simulink library "ddm"  (R2021b)
settings: Solver=VariableStepAuto  StartTime=0.0  StopTime=10.0  RelTol=1e-3
undefined symbols (not defined in the file or in its folder): ADDM_FrTMTqDev_X_Nm, ADDM_RrTMTqDev_X_Nm, ENUM_ADASACCSTA_ERROR, ENUM_ADASACCSTA_OFF, ENUM_ADASACCSTA_STANDBY, ENUM_ALLOWMOV_ALLOWREADY, ENUM_APS, ENUM_BRKSTA_ERROR, ENUM_BRKSTA_OFF, ENUM_BRKSTA_ON, ENUM_BRKSW_INVALID, ENUM_BRKSW_OFF, ENUM_BRKSW_ON, ENUM_CHGPREACTERRSTA_OBCPRE, ENUM_DCDCFAULTSTA_ANYFAULTLV1, ENUM_DCDCFAULTSTA_ANYFAULTLV2, ENUM_DRIVETRAIN_AWD, ENUM_DRIVETRAIN_FWD, ENUM_DRIVETRAIN_RWD, ENUM_EDUDRTSTA_NORMAL, ENUM_EPBSTA_APPLIED, ENUM_EPBSTA_RELEASED, ENUM_GEARACTUALPOSN_INVALID, ENUM_GEARACTUALPOSN_P, ENUM_HVBATTREADYPRE_READY, ENUM_MCUWARN_LV0, ENUM_MCUWARN_LV1, ENUM_MCUWARN_LV2, ENUM_MCUWARN_LV3, ENUM_MCUWARN_NOERROR, ENUM_OBCFAULTSTA_ANYFAULT, ENUM_PAS_R2F2, ENUM_PDFAULT_BATTPDFAIL, ENUM_PDFAULT_DCDCDISABLE, ENUM_PDFAULT_MCUDISABLE, ENUM_PDFAULT_MCUDISCHRG, ENUM_POWERSTA_OFF, ENUM_POWERSTA_ON, ENUM_POWERSTA_READY, ENUM_POWERSTA_STANDBY, ENUM_PRESSINDI_LOW, ENUM_PUFAULT_BATTUPFAIL, ENUM_PUFAULT_DCDCENABLEFAIL, ENUM_PUFAULT_PRECHRGCHKFAIL, ENUM_PUFAULT_SAFETYCHKFAIL, ENUM_PUSTATE_COMPLETED, ENUM_PWRSTASW_OFF, ENUM_PWRSTASW_OFFA, ENUM_PWRSTASW_OFFCHVCHRG, ENUM_PWRSTASW_OFFCLVCHRG, ENUM_PWRSTASW_ON, ENUM_PWRSTASW_ONHVCHRG, ENUM_PWRSTASW_READY, ENUM_PWRSTASW_STANDBY, ENUM_SHIFTCOMMAND_P, ENUM_SHIFTERERRSTA_PBUTTONFAILURE, ENUM_VEHMALFUNLV_2ND, ENUM_VEHMALFUNLV_3RD, ENUM_VEHMALFUNLV_4TH, ENUM_VEHMALFUNLV_NORMAL ... (+459)
libraries: hcu_lib x521, $bdroot x5, simulink x3
(part 8 of 25)

== system ddm/DDM/DDM/APM/Subsystem9 ==
  USSSta_flg : Inport
  VPMM_SysPwrSta_enum : Inport  Port=2
  VAPM_SNSRLayout_enum : Inport  Port=3
  Constant1 : Constant  Value=ENUM_PWRSTASW_READY
  Constant17 : Constant  Value=ENUM_PWRSTASW_READY
  Constant2 : Constant  Value=ENUM_PWRSTASW_ON
  Constant25 : Constant  Value=FALSE
  Constant3 : Constant  Value=ENUM_PWRSTASW_ON
  Constant5 : Constant  Value=ENUM_APS
  Equal{1..3,5..6} (5 alike) : RelationalOperator  Operator===  OutDataTypeStr=boolean  RndMeth=Simplest
  Logical Operator1 : Logic  Operator=NOT  AllPortsSameDT=off  OutDataTypeStr=boolean
  Logical Operator13 : Logic  Operator=OR  AllPortsSameDT=off  OutDataTypeStr=boolean
  Logical Operator2 : Logic  AllPortsSameDT=off  OutDataTypeStr=boolean
  Logical Operator3 : Logic  Operator=OR  AllPortsSameDT=off  OutDataTypeStr=boolean
  Logical Operator4 : Logic  AllPortsSameDT=off  OutDataTypeStr=boolean
  Switch2 : Switch  Criteria=u2 ~= 0
  Pass_flg : Outport
  CFS_flg : Outport  Port=2
  wires:
  [VPMM_SysPwrSta_enum] -> Equal2/1
  Equal6/1 -> Logical Operator13/1
  Constant17/1 -> Equal2/2
  Constant3/1 -> Equal6/2
  Equal2/1 -> Logical Operator13/2
  [VPMM_SysPwrSta_enum] -> Equal6/1
  Logical Operator13/1 -> Logical Operator2/1
  Logical Operator1/1 -> Logical Operator2/2
  Logical Operator2/1 -> Pass_flg/1
  Logical Operator3/1 -> Logical Operator4/2
  [VPMM_SysPwrSta_enum] -> Equal3/1
  Equal1/1 -> Logical Operator3/2
  Constant2/1 -> Equal3/2
  Constant1/1 -> Equal1/2
  Equal3/1 -> Logical Operator3/1
  [VPMM_SysPwrSta_enum] -> Equal1/1
  Switch2/1 -> Logical Operator4/1, Logical Operator1/1
  Logical Operator4/1 -> CFS_flg/1
  VPMM_SysPwrSta_enum/1 -> [VPMM_SysPwrSta_enum]
  Constant5/1 -> Equal5/2
  VAPM_SNSRLayout_enum/1 -> Equal5/1
  Equal5/1 -> Switch2/2
  Constant25/1 -> Switch2/3
  USSSta_flg/1 -> Switch2/1

== system ddm/DDM/DDM/Enabled Subsystem/Subsystem ==
  KDDM_DTCClockerMax_cnt : Inport
  Trigger : TriggerPort  VariantControl=(inherit)  ZeroCross=off  PortDimensions=1
  Add : Sum
  Constant : Constant  Value=ZERO_INT
  Constant1 : Constant  Value=ONE_INT
  Data Type Conversion : DataTypeConversion  OutDataTypeStr=uint8
  Delay : Delay  DelayLength=1
  Relational Operator : RelationalOperator  OutDataTypeStr=boolean  RndMeth=Simplest
  Switch : Switch  Criteria=u2 > Threshold
  VDDM_DTCCounter_cnt : Outport
  wires:
  Data Type Conversion/1 -> [VDDM_DTCCounter_cnt]
  Switch/1 -> Data Type Conversion/1, Delay/1
  [VDDM_DTCCounter_cnt] -> VDDM_DTCCounter_cnt/1
  Constant1/1 -> Add/1
  Delay/1 -> Relational Operator/1, Add/2
  Add/1 -> Switch/3
  [KDDM_DTCClockerMax_cnt] -> Relational Operator/2
  Constant/1 -> Switch/1
  Relational Operator/1 -> Switch/2
  KDDM_DTCClockerMax_cnt/1 -> [KDDM_DTCClockerMax_cnt]

== system ddm/DDM/DDM/PMM/Brake switch signal abnormal ==
  task_time_s : Inport
  VPMM_PowerSta_enum : Inport  Port=2
  VINP_BrakeSWGPIO_flg : Inport  Port=3
  VINP_BrakeLampSW_flg : Inport  Port=4
  VDDM_ESC5NoComCFS_flg : Inport  Port=5
  VDDM_ESC5RCErrCFS_flg : Inport  Port=6
  VDDM_ESC5CSErrCFS_flg : Inport  Port=7
  VINP_DrStdAErrSta_enum : Inport  Port=8
  VINP_BrkSWSta_flg : Inport  Port=9
  VINP_BrkPedalPosSta_enum : Inport  Port=10
  VINP_BrkPedalPos_pct : Inport  Port=11
  DTC_clear_request : Inport  Port=12
  Brake switch signal abnormal : Subsystem
  Brake switch signal abnormal and no backup signal : Subsystem
  Constant : Constant  Value=TRUE
  Constant1 : Constant  Value=ENUM_BRKSTA_ERROR
  Constant2 : Constant  Value=ENUM_BRKSTA_ON
  Constant3 : Constant  Value=ENUM_BRKSTA_OFF
  Constant4 : Constant  Value=FALSE
  Constant5 : Constant  Value=ENUM_BRKSTA_ERROR
  Constant6 : Constant  Value=ENUM_BRKSTA_ON
  Constant7 : Constant  Value=ENUM_BRKSTA_OFF
  Constant8 : Constant  Value=KDDM_BrkPedalPos_pct
  Equal : RelationalOperator  Operator===  OutDataTypeStr=boolean  RndMeth=Simplest
  Equal1 : RelationalOperator  Operator===  OutDataTypeStr=boolean  RndMeth=Simplest
  Equal2 : RelationalOperator  OutDataTypeStr=boolean  RndMeth=Simplest
  Logical Operator : Logic  Operator=OR  Inputs=4  AllPortsSameDT=off  OutDataTypeStr=boolean
  Logical Operator1 : Logic  Operator=OR  Inputs=4  AllPortsSameDT=off  OutDataTypeStr=boolean
  Subsystem : Subsystem
  Switch{,1..3} (4 alike) : Switch  Criteria=u2 > Threshold
  Terminator : Terminator
  VDDM_BrkSWErrDTC_raw32 : Outport
  VDDM_BrkSWNoBacDTC_raw32 : Outport  Port=2
  VDDM_BrakeSW_enum : Outport  Port=3
  VDDM_CANBrkSW2Sta_enum : Outport  Port=4
  VDDM_BrkPedalPosSta_enum : Outport  Port=5
  VDDM_BrkSWErrCFS_flg : Outport  Port=6
  VDDM_BrkSWNoBacCFS_flg : Outport  Port=7
  VDDM_VCUBrkSWSta_enum : Outport  Port=8
  VDDM_EDriveSysErrBrake_flg : Outport  Port=9
  wires:
  [VDDM_BrkSWErr_flg] -> Brake switch signal abnormal/3(BrkSWErr)
  Subsystem/3(BrkSWPass) -> Terminator/1  "VDDM_BrkSWPass_flg"
  Subsystem/2(BrkSWNoBac) -> [VDDM_BrkSWNoBac_flg]  "VDDM_BrkSWNoBac_flg"
  Subsystem/4(VDDM_BrakeSW_enum) -> [VDDM_BrakeSW_enum], [VDDM_VCUBrkSWSta_enum]  "VDDM_BrakeSW_enum"
  Subsystem/1(BrkSWErr) -> [VDDM_BrkSWErr_flg]  "VDDM_BrkSWErr_flg"
  VINP_BrakeLampSW_flg/1 -> Subsystem/3(Brake_Stop_Lamp)
  VINP_BrakeSWGPIO_flg/1 -> Subsystem/2(BrakeSW)
  [VDDM_BrkPedalPosSta_enum] -> Subsystem/4(BrkPedalPos_enum)
  [VDDM_CANBrkSW2Sta_enum] -> Subsystem/1(VDDM_CANBSW2S_enum)
  [DTC_clear_request] -> Brake switch signal abnormal/4(DTC_clear_request)
  DTC_clear_request/1 -> [DTC_clear_request]
  [VDDM_BrakeSW_enum] -> VDDM_BrakeSW_enum/1
  [VDDM_CANBrkSW2Sta_enum] -> VDDM_CANBrkSW2Sta_enum/1
  [VDDM_BrkPedalPosSta_enum] -> VDDM_BrkPedalPosSta_enum/1
  Switch2/1 -> [VDDM_BrkPedalPosSta_enum]  "VDDM_BrkPedalPosSta_enum"
  Switch/1 -> [VDDM_CANBrkSW2Sta_enum]  "VDDM_CANBrkSW2Sta_enum"
  Brake switch signal abnormal and no backup signal/1(VDDM_BrkSWNoBacDTC_raw32) -> VDDM_BrkSWNoBacDTC_raw32/1
  Brake switch signal abnormal/1(VDDM_BrkSWErrDTC_raw32) -> VDDM_BrkSWErrDTC_raw32/1
  Equal2/1 -> Switch3/2
  Constant8/1 -> Equal2/2
  VINP_BrkPedalPosSta_enum/1 -> Equal1/1
  Constant4/1 -> Equal1/2
  Equal1/1 -> Logical Operator1/4
  Switch3/1 -> Switch2/3
  Logical Operator1/1 -> Switch2/2
  Constant5/1 -> Switch2/1
  Constant6/1 -> Switch3/1
  Constant7/1 -> Switch3/3
  Constant3/1 -> Switch1/3
  Constant2/1 -> Switch1/1
  VINP_BrkSWSta_flg/1 -> Switch1/2
  Constant1/1 -> Switch/1
  Logical Operator/1 -> Switch/2
  Switch1/1 -> Switch/3
  Equal/1 -> Logical Operator/4
  Constant/1 -> Equal/2
  VINP_DrStdAErrSta_enum/1 -> Equal/1
  task_time_s/1 -> [task_time_s]
  VPMM_PowerSta_enum/1 -> [VPMM_PowerSta_enum]
  [task_time_s] -> Brake switch signal abnormal/1(task_time_s)
  Brake switch signal abnormal/2(VDDM_BrkSWErrCFS_flg) -> [VDDM_BrkSWErrCFS_flg]
  [VPMM_PowerSta_enum] -> Brake switch signal abnormal/2(VPMM_PowerSta_enum)
  Brake switch signal abnormal and no backup signal/2(VDDM_BrkSWNoBacCFS_flg) -> [VDDM_BrkSWNoBacCFS_flg], [VDDM_EDriveSysErrBrake_flg]
  [DTC_clear_request] -> Brake switch signal abnormal and no backup signal/4(DTC_clear_request)
  [VDDM_BrkSWNoBac_flg] -> Brake switch signal abnormal and no backup signal/3(BrkSWNoBac)
  [VPMM_PowerSta_enum] -> Brake switch signal abnormal and no backup signal/2(VPMM_PowerSta_enum)
  [task_time_s] -> Brake switch signal abnormal and no backup signal/1(task_time_s)
  [VDDM_BrkSWErrCFS_flg] -> VDDM_BrkSWErrCFS_flg/1
  [VDDM_BrkSWNoBacCFS_flg] -> VDDM_BrkSWNoBacCFS_flg/1
  [VDDM_VCUBrkSWSta_enum] -> VDDM_VCUBrkSWSta_enum/1  "VDDM_VCUBrkSWSta_enum"
  [VDDM_EDriveSysErrBrake_flg] -> VDDM_EDriveSysErrBrake_flg/1
  VDDM_ESC5NoComCFS_flg/1 -> [VDDM_ESC5NoComCFS_flg]
  VDDM_ESC5RCErrCFS_flg/1 -> [VDDM_ESC5RCErrCFS_flg]
  VDDM_ESC5CSErrCFS_flg/1 -> [VDDM_ESC5CSErrCFS_flg]
  [VDDM_ESC5NoComCFS_flg] -> Logical Operator/1
  [VDDM_ESC5RCErrCFS_flg] -> Logical Operator/2
  [VDDM_ESC5CSErrCFS_flg] -> Logical Operator/3
  [VDDM_ESC5CSErrCFS_flg] -> Logical Operator1/3
  [VDDM_ESC5RCErrCFS_flg] -> Logical Operator1/2
  [VDDM_ESC5NoComCFS_flg] -> Logical Operator1/1
  VINP_BrkPedalPos_pct/1 -> [VINP_BrkPedalPos_pct]
  [VINP_BrkPedalPos_pct] -> Equal2/1
  [VINP_BrkPedalPos_pct] -> Brake switch signal abnormal/5(VINP_BrkPedalPos_pct)
  [VINP_BrkPedalPos_pct] -> Brake switch signal abnormal and no backup signal/5(VINP_BrkPedalPos_pct)

== system ddm/DDM/DDM/PMM/Comm err ==
  note: CAN3 BMS6
  note: CAN3 BMS1
  note: CAN3 CCU1
  note: CAN3 CCU2
  note: CAN1 ABM1
  task_time_s : Inport
  VPMM_PowerSta_enum : Inport  Port=2
  VPMM_PwrStaSW_enum : Inport  Port=3
  VDDM_C3BMS6RCChk_flg : Inport  Port=4
  VDDM_C3BMS6CSChk_flg : Inport  Port=5
  VDDM_C3BMS6LCChk_flg : Inport  Port=6
  VDDM_C3BMS1RCChk_flg : Inport  Port=7
  VDDM_C3BMS1CSChk_flg : Inport  Port=8
  VDDM_C3BMS1LCChk_flg : Inport  Port=9
  VDDM_C3CCU1RCChk_flg : Inport  Port=10
  VDDM_C3CCU1CSChk_flg : Inport  Port=11
  VDDM_C3CCU1LCChk_flg : Inport  Port=12
  VDDM_C3CCU2RCChk_flg : Inport  Port=13
  VDDM_C3CCU2CSChk_flg : Inport  Port=14
  VDDM_C3CCU2LCChk_flg : Inport  Port=15
  VDDM_C1ABM1RCChk_flg : Inport  Port=16
  VDDM_C1ABM1CSChk_flg : Inport  Port=17
  VDDM_C1ABM1LCChk_flg : Inport  Port=18
  No_CAN3_BUS_OFF : Inport  Port=19
  No_CAN1_BUS_OFF : Inport  Port=20
  DTC_clear_request : Inport  Port=21
  OR : Logic  Operator=OR  Inputs=3  AllPortsSameDT=off  OutDataTypeStr=boolean
  The CAN signal between VCU and ABM1 is discontinuous : Subsystem
  The CAN signal between VCU and ABM1 is incomplete : Subsystem
  The CAN signal between VCU and BMS1 is discontinuous : Subsystem
  The CAN signal between VCU and BMS1 is incomplete : Subsystem
  The CAN signal between VCU and BMS6 is discontinuous : Subsystem
  The CAN signal between VCU and BMS6 is incomplete : Subsystem
  The CAN signal between VCU and CCU1 is discontinuous : Subsystem
  The CAN signal between VCU and CCU1 is incomplete : Subsystem
  The CAN signal between VCU and CCU2 is discontinuous : Subsystem
  The CAN signal between VCU and CCU2 is incomplete : Subsystem
  VCU lost communication with ABM1 : Subsystem
  VCU lost communication with BMS1 : Subsystem
  VCU lost communication with BMS6 : Subsystem
  VCU lost communication with CCU1 : Subsystem
  VCU lost communication with CCU2 : Subsystem
  VDDM_C3BMS6RCDTC_raw32 : Outport
  VDDM_C3BMS6CSDTC_raw32 : Outport  Port=2
  VDDM_C3BMS6LCDTC_raw32 : Outport  Port=3
  VDDM_C3BMS1RCDTC_raw32 : Outport  Port=4
  VDDM_C3BMS1CSDTC_raw32 : Outport  Port=5
  VDDM_C3BMS1LCDTC_raw32 : Outport  Port=6
  VDDM_C3CCU1RCDTC_raw32 : Outport  Port=7
  VDDM_C3CCU1CSDTC_raw32 : Outport  Port=8
  VDDM_C3CCU1LCDTC_raw32 : Outport  Port=9
  VDDM_C3CCU2RCDTC_raw32 : Outport  Port=10
  VDDM_C3CCU2CSDTC_raw32 : Outport  Port=11
  VDDM_C3CCU2LCDTC_raw32 : Outport  Port=12
  VDDM_C1ABM1RCDTC_raw32 : Outport  Port=13
  VDDM_C1ABM1CSDTC_raw32 : Outport  Port=14
  VDDM_C1ABM1LCDTC_raw32 : Outport  Port=15
  VDDM_C3BMS6RCCFS_flg : Outport  Port=16
  VDDM_C3BMS6CSCFS_flg : Outport  Port=17
  VDDM_C3BMS6LCCFS_flg : Outport  Port=18
  VDDM_C3BMS1RCCFS_flg : Outport  Port=19
  VDDM_C3BMS1CSCFS_flg : Outport  Port=20
  VDDM_C3BMS1LCCFS_flg : Outport  Port=21
  VDDM_C3CCU1RCCFS_flg : Outport  Port=22
  VDDM_C3CCU1CSCFS_flg : Outport  Port=23
  VDDM_C3CCU1LCCFS_flg : Outport  Port=24
  VDDM_C3CCU2RCCFS_flg : Outport  Port=25
  VDDM_C3CCU2CSCFS_flg : Outport  Port=26
  VDDM_C3CCU2LCCFS_flg : Outport  Port=27
  VDDM_C1ABM1RCCFS_flg : Outport  Port=28
  VDDM_C1ABM1CSCFS_flg : Outport  Port=29
  VDDM_C1ABM1LCCFS_flg : Outport  Port=30
  VDDM_EDriveSysErrABMCAN_flg : Outport  Port=31
  wires:
  The CAN signal between VCU and CCU2 is discontinuous/2(VDDM_C3CCU2RCCFS_flg) -> VDDM_C3CCU2RCCFS_flg/1
  The CAN signal between VCU and CCU2 is incomplete/2(VDDM_C3CCU2CSCFS_flg) -> VDDM_C3CCU2CSCFS_flg/1
  The CAN signal between VCU and BMS6 is discontinuous/2(VDDM_C3BMS6RCCFS_flg) -> VDDM_C3BMS6RCCFS_flg/1
  The CAN signal between VCU and BMS6 is incomplete/2(VDDM_C3BMS6CSCFS_flg) -> VDDM_C3BMS6CSCFS_flg/1
  The CAN signal between VCU and CCU1 is discontinuous/1(VDDM_C3CCU1RCDTC_raw32) -> VDDM_C3CCU1RCDTC_raw32/1
  VCU lost communication with BMS6/1(VDDM_C3BMS6LCDTC_raw32) -> VDDM_C3BMS6LCDTC_raw32/1
  VCU lost communication with ABM1/1(VDDM_C1ABM1LCDTC_raw32) -> VDDM_C1ABM1LCDTC_raw32/1
  The CAN signal between VCU and ABM1 is incomplete/1(VDDM_C1ABM1CSDTC_raw32) -> VDDM_C1ABM1CSDTC_raw32/1
  The CAN signal between VCU and ABM1 is discontinuous/1(VDDM_C1ABM1RCDTC_raw32) -> VDDM_C1ABM1RCDTC_raw32/1
  VCU lost communication with CCU2/1(VDDM_C3CCU2LCDTC_raw32) -> VDDM_C3CCU2LCDTC_raw32/1
  The CAN signal between VCU and CCU2 is incomplete/1(VDDM_C3CCU2CSDTC_raw32) -> VDDM_C3CCU2CSDTC_raw32/1
  The CAN signal between VCU and CCU2 is discontinuous/1(VDDM_C3CCU2RCDTC_raw32) -> VDDM_C3CCU2RCDTC_raw32/1
  VCU lost communication with CCU1/1(VDDM_C3CCU1LCDTC_raw32) -> VDDM_C3CCU1LCDTC_raw32/1
  The CAN signal between VCU and CCU1 is incomplete/1(VDDM_C3CCU1CSDTC_raw32) -> VDDM_C3CCU1CSDTC_raw32/1
  VCU lost communication with BMS1/1(VDDM_C3BMS1LCDTC_raw32) -> VDDM_C3BMS1LCDTC_raw32/1
  The CAN signal between VCU and BMS1 is incomplete/1(VDDM_C3BMS1CSDTC_raw32) -> VDDM_C3BMS1CSDTC_raw32/1
  The CAN signal between VCU and BMS1 is discontinuous/1(VDDM_C3BMS1RCDTC_raw32) -> VDDM_C3BMS1RCDTC_raw32/1
  The CAN signal between VCU and BMS6 is incomplete/1(VDDM_C3BMS6CSDTC_raw32) -> VDDM_C3BMS6CSDTC_raw32/1
  The CAN signal between VCU and BMS6 is discontinuous/1(VDDM_C3BMS6RCDTC_raw32) -> VDDM_C3BMS6RCDTC_raw32/1
  DTC_clear_request/1 -> [DTC_clear_request]
  No_CAN1_BUS_OFF/1 -> [No_CAN1_BUS_OFF]
  No_CAN3_BUS_OFF/1 -> [No_CAN3_BUS_OFF]
  OR/1 -> VDDM_EDriveSysErrABMCAN_flg/1
  [VDDM_EDriveSysErrABMLC_flg] -> OR/3
  [VDDM_EDriveSysErrABMRC_flg] -> OR/1
  [VDDM_EDriveSysErrABMCS_flg] -> OR/2
  VCU lost communication with ABM1/3(LC_EDriveSysErr_VCUErr_flg) -> [VDDM_EDriveSysErrABMLC_flg]
  [DTC_clear_request] -> VCU lost communication with ABM1/6(DTC_clear_request)
  [No_CAN1_BUS_OFF] -> VCU lost communication with ABM1/5(No_CAN1_BUS_OFF)
  The CAN signal between VCU and ABM1 is incomplete/2(CS_EDriveSysErr_VCUErr_flg) -> [VDDM_EDriveSysErrABMCS_flg]
  The CAN signal between VCU and ABM1 is discontinuous/2(RC_EDriveSysErr_VCUErr_flg) -> [VDDM_EDriveSysErrABMRC_flg]
  [DTC_clear_request] -> The CAN signal between VCU and ABM1 is incomplete/7(DTC_clear_request)
  [No_CAN1_BUS_OFF] -> The CAN signal between VCU and ABM1 is incomplete/6(No_CAN1_BUS_OFF)
  [DTC_clear_request] -> The CAN signal between VCU and ABM1 is discontinuous/7(DTC_clear_request)
  [No_CAN1_BUS_OFF] -> The CAN signal between VCU and ABM1 is discontinuous/6(No_CAN1_BUS_OFF)
  [DTC_clear_request] -> VCU lost communication with CCU2/6(DTC_clear_request)
  [No_CAN3_BUS_OFF] -> VCU lost communication with CCU2/5(No_CAN3_BUS_OFF)
  [DTC_clear_request] -> The CAN signal between VCU and CCU2 is incomplete/7(DTC_clear_request)
  [No_CAN3_BUS_OFF] -> The CAN signal between VCU and CCU2 is incomplete/6(No_CAN3_BUS_OFF)
  [DTC_clear_request] -> The CAN signal between VCU and CCU2 is discontinuous/7(DTC_clear_request)
  [No_CAN3_BUS_OFF] -> The CAN signal between VCU and CCU2 is discontinuous/6(No_CAN3_BUS_OFF)
  [DTC_clear_request] -> VCU lost communication with CCU1/6(DTC_clear_request)
  [No_CAN3_BUS_OFF] -> VCU lost communication with CCU1/5(No_CAN3_BUS_OFF)
  [DTC_clear_request] -> The CAN signal between VCU and CCU1 is incomplete/7(DTC_clear_request)
  [No_CAN3_BUS_OFF] -> The CAN signal between VCU and CCU1 is incomplete/6(No_CAN3_BUS_OFF)
  [DTC_clear_request] -> The CAN signal between VCU and CCU1 is discontinuous/7(DTC_clear_request)
  [No_CAN3_BUS_OFF] -> The CAN signal between VCU and CCU1 is discontinuous/6(No_CAN3_BUS_OFF)
  [DTC_clear_request] -> VCU lost communication with BMS1/6(DTC_clear_request)
  [No_CAN3_BUS_OFF] -> VCU lost communication with BMS1/5(No_CAN3_BUS_OFF)
  [DTC_clear_request] -> The CAN signal between VCU and BMS1 is incomplete/7(DTC_clear_request)
  [No_CAN3_BUS_OFF] -> The CAN signal between VCU and BMS1 is incomplete/6(No_CAN3_BUS_OFF)
  [VDDM_C3BMS1LCCFS_flg] -> The CAN signal between VCU and BMS1 is discontinuous/5(VDDM_C3BMS1LCCFS_flg)
  [DTC_clear_request] -> The CAN signal between VCU and BMS1 is discontinuous/7(DTC_clear_request)
  [DTC_clear_request] -> VCU lost communication with BMS6/6(DTC_clear_request)
  [No_CAN3_BUS_OFF] -> VCU lost communication with BMS6/5(No_CAN3_BUS_OFF)
  [VDDM_C3BMS6LCCFS_flg] -> The CAN signal between VCU and BMS6 is incomplete/5(VDDM_C3BMS6LCCFS_flg)
  [VDDM_C3BMS6LCCFS_flg] -> The CAN signal between VCU and BMS6 is discontinuous/5(VDDM_C3BMS6LCCFS_flg)
  [DTC_clear_request] -> The CAN signal between VCU and BMS6 is incomplete/7(DTC_clear_request)
  [DTC_clear_request] -> The CAN signal between VCU and BMS6 is discontinuous/7(DTC_clear_request)
  VDDM_C3BMS6LCChk_flg/1 -> VCU lost communication with BMS6/4(VDDM_C3BMS6LCChk_flg)
  VDDM_C3BMS6CSChk_flg/1 -> The CAN signal between VCU and BMS6 is incomplete/4(VDDM_C3BMS6CSChk_flg)
  VDDM_C3BMS6RCChk_flg/1 -> The CAN signal between VCU and BMS6 is discontinuous/4(VDDM_C3BMS6RCChk_flg)
  task_time_s/1 -> [task_time_s]
  VPMM_PwrStaSW_enum/1 -> [VPMM_PwrStaSW_enum]
  VPMM_PowerSta_enum/1 -> [VPMM_PowerSta_enum]
  VDDM_C3CCU2RCChk_flg/1 -> The CAN signal between VCU and CCU2 is discontinuous/4(VDDM_C3CCU2RCChk_flg)
  VDDM_C3CCU2LCChk_flg/1 -> VCU lost communication with CCU2/4(VDDM_C3CCU2LCChk_flg)
  VDDM_C3CCU1CSChk_flg/1 -> The CAN signal between VCU and CCU1 is incomplete/4(VDDM_C3CCU1CSChk_flg)
  VDDM_C3BMS1CSChk_flg/1 -> The CAN signal between VCU and BMS1 is incomplete/4(VDDM_C3BMS1CSChk_flg)
  VDDM_C1ABM1CSChk_flg/1 -> The CAN signal between VCU and ABM1 is incomplete/4(VDDM_C1ABM1CSChk_flg)
  VDDM_C1ABM1RCChk_flg/1 -> The CAN signal between VCU and ABM1 is discontinuous/4(VDDM_C1ABM1RCChk_flg)
  VDDM_C3CCU1RCChk_flg/1 -> The CAN signal between VCU and CCU1 is discontinuous/4(VDDM_C3CCU1RCChk_flg)
  VDDM_C3CCU1LCChk_flg/1 -> VCU lost communication with CCU1/4(VDDM_C3CCU1LCChk_flg)
  VDDM_C3BMS1RCChk_flg/1 -> The CAN signal between VCU and BMS1 is discontinuous/4(VDDM_C3BMS1RCChk_flg)
  VDDM_C3CCU2CSChk_flg/1 -> The CAN signal between VCU and CCU2 is incomplete/4(VDDM_C3CCU2CSChk_flg)
  [VPMM_PowerSta_enum] -> The CAN signal between VCU and ABM1 is discontinuous/2(VPMM_PowerSta_enum)
  [task_time_s] -> The CAN signal between VCU and ABM1 is discontinuous/1(task_time_s)
  [VDDM_C1ABM1LCCFS_flg] -> The CAN signal between VCU and ABM1 is incomplete/5(VDDM_C1ABM1LCCFS_flg)
  [VPMM_PwrStaSW_enum] -> The CAN signal between VCU and CCU2 is incomplete/3(VPMM_PwrStaSW_enum)
  [VPMM_PowerSta_enum] -> The CAN signal between VCU and ABM1 is incomplete/2(VPMM_PowerSta_enum)
  [VPMM_PowerSta_enum] -> VCU lost communication with CCU2/2(VPMM_PowerSta_enum)
  [task_time_s] -> The CAN signal between VCU and CCU2 is incomplete/1(task_time_s)
  [VPMM_PwrStaSW_enum] -> The CAN signal between VCU and CCU2 is discontinuous/3(VPMM_PwrStaSW_enum)
  VCU lost communication with BMS6/2(VDDM_C3BMS6LCCFS_flg) -> [VDDM_C3BMS6LCCFS_flg], VDDM_C3BMS6LCCFS_flg/1
  [VPMM_PowerSta_enum] -> The CAN signal between VCU and CCU1 is discontinuous/2(VPMM_PowerSta_enum)
  [VDDM_C3CCU1LCCFS_flg] -> The CAN signal between VCU and CCU1 is incomplete/5(VDDM_C3CCU1LCCFS_flg)
  [VPMM_PwrStaSW_enum] -> VCU lost communication with CCU1/3(VPMM_PwrStaSW_enum)
  [VPMM_PowerSta_enum] -> VCU lost communication with CCU1/2(VPMM_PowerSta_enum)
  [VPMM_PwrStaSW_enum] -> The CAN signal between VCU and CCU1 is incomplete/3(VPMM_PwrStaSW_enum)
  [VPMM_PwrStaSW_enum] -> The CAN signal between VCU and CCU1 is discontinuous/3(VPMM_PwrStaSW_enum)
  [VPMM_PwrStaSW_enum] -> The CAN signal between VCU and BMS6 is discontinuous/3(VPMM_PwrStaSW_enum)
  [task_time_s] -> The CAN signal between VCU and CCU1 is discontinuous/1(task_time_s)
  [VPMM_PowerSta_enum] -> The CAN signal between VCU and CCU1 is incomplete/2(VPMM_PowerSta_enum)
  [No_CAN3_BUS_OFF] -> The CAN signal between VCU and BMS6 is discontinuous/6(No_CAN3_BUS_OFF)
  VCU lost communication with CCU1/2(VDDM_C3CCU1LCCFS_flg) -> [VDDM_C3CCU1LCCFS_flg], VDDM_C3CCU1LCCFS_flg/1
  [No_CAN3_BUS_OFF] -> The CAN signal between VCU and BMS1 is discontinuous/6(No_CAN3_BUS_OFF)
  [task_time_s] -> VCU lost communication with BMS1/1(task_time_s)
  [VPMM_PowerSta_enum] -> VCU lost communication with BMS6/2(VPMM_PowerSta_enum)
  [VPMM_PwrStaSW_enum] -> The CAN signal between VCU and BMS1 is incomplete/3(VPMM_PwrStaSW_enum)
  [VPMM_PowerSta_enum] -> The CAN signal between VCU and CCU2 is incomplete/2(VPMM_PowerSta_enum)
  [task_time_s] -> VCU lost communication with CCU1/1(task_time_s)
  [VDDM_C3BMS1LCCFS_flg] -> The CAN signal between VCU and BMS1 is incomplete/5(VDDM_C3BMS1LCCFS_flg)
  [VPMM_PowerSta_enum] -> The CAN signal between VCU and BMS1 is incomplete/2(VPMM_PowerSta_enum)
  VDDM_C3BMS1LCChk_flg/1 -> VCU lost communication with BMS1/4(VDDM_C3BMS1LCChk_flg)
  [task_time_s] -> The CAN signal between VCU and ABM1 is incomplete/1(task_time_s)
  [VPMM_PowerSta_enum] -> The CAN signal between VCU and BMS1 is discontinuous/2(VPMM_PowerSta_enum)
  [No_CAN3_BUS_OFF] -> The CAN signal between VCU and BMS6 is incomplete/6(No_CAN3_BUS_OFF)
  [VPMM_PwrStaSW_enum] -> VCU lost communication with BMS1/3(VPMM_PwrStaSW_enum)
  [VDDM_C3CCU2LCCFS_flg] -> The CAN signal between VCU and CCU2 is discontinuous/5(VDDM_C3CCU2LCCFS_flg)
  [VPMM_PowerSta_enum] -> The CAN signal between VCU and BMS6 is incomplete/2(VPMM_PowerSta_enum)
  [VDDM_C3CCU1LCCFS_flg] -> The CAN signal between VCU and CCU1 is discontinuous/5(VDDM_C3CCU1LCCFS_flg)
  [VPMM_PwrStaSW_enum] -> The CAN signal between VCU and BMS1 is discontinuous/3(VPMM_PwrStaSW_enum)
  [task_time_s] -> The CAN signal between VCU and BMS1 is discontinuous/1(task_time_s)
  [VPMM_PowerSta_enum] -> VCU lost communication with BMS1/2(VPMM_PowerSta_enum)
  [VPMM_PowerSta_enum] -> The CAN signal between VCU and CCU2 is discontinuous/2(VPMM_PowerSta_enum)
  VCU lost communication with BMS1/2(VDDM_C3BMS1LCCFS_flg) -> [VDDM_C3BMS1LCCFS_flg], VDDM_C3BMS1LCCFS_flg/1
  [task_time_s] -> The CAN signal between VCU and CCU1 is incomplete/1(task_time_s)
  [VDDM_C1ABM1LCCFS_flg] -> The CAN signal between VCU and ABM1 is discontinuous/5(VDDM_C1ABM1LCCFS_flg)
  [task_time_s] -> The CAN signal between VCU and BMS6 is incomplete/1(task_time_s)
  VDDM_C1ABM1LCChk_flg/1 -> VCU lost communication with ABM1/4(VDDM_C1ABM1LCChk_flg)
  [VPMM_PwrStaSW_enum] -> The CAN signal between VCU and ABM1 is incomplete/3(VPMM_PwrStaSW_enum)
  VCU lost communication with ABM1/2(VDDM_C1ABM1LCCFS_flg) -> [VDDM_C1ABM1LCCFS_flg], VDDM_C1ABM1LCCFS_flg/1
  [task_time_s] -> VCU lost communication with CCU2/1(task_time_s)
  [VPMM_PowerSta_enum] -> The CAN signal between VCU and BMS6 is discontinuous/2(VPMM_PowerSta_enum)
  [VPMM_PwrStaSW_enum] -> The CAN signal between VCU and ABM1 is discontinuous/3(VPMM_PwrStaSW_enum)
  [VPMM_PowerSta_enum] -> VCU lost communication with ABM1/2(VPMM_PowerSta_enum)
  [VPMM_PwrStaSW_enum] -> VCU lost communication with BMS6/3(VPMM_PwrStaSW_enum)
  [task_time_s] -> The CAN signal between VCU and BMS1 is incomplete/1(task_time_s)
  [task_time_s] -> VCU lost communication with ABM1/1(task_time_s)
  VCU lost communication with CCU2/2(VDDM_C3CCU2LCCFS_flg) -> [VDDM_C3CCU2LCCFS_flg], VDDM_C3CCU2LCCFS_flg/1
  [VPMM_PwrStaSW_enum] -> VCU lost communication with ABM1/3(VPMM_PwrStaSW_enum)
  [task_time_s] -> The CAN signal between VCU and BMS6 is discontinuous/1(task_time_s)
  [task_time_s] -> The CAN signal between VCU and CCU2 is discontinuous/1(task_time_s)
  [task_time_s] -> VCU lost communication with BMS6/1(task_time_s)
  [VPMM_PwrStaSW_enum] -> VCU lost communication with CCU2/3(VPMM_PwrStaSW_enum)
  [VPMM_PwrStaSW_enum] -> The CAN signal between VCU and BMS6 is incomplete/3(VPMM_PwrStaSW_enum)
  [VDDM_C3CCU2LCCFS_flg] -> The CAN signal between VCU and CCU2 is incomplete/5(VDDM_C3CCU2LCCFS_flg)
  The CAN signal between VCU and BMS1 is discontinuous/2(VDDM_C3BMS1RCCFS_flg) -> VDDM_C3BMS1RCCFS_flg/1
  The CAN signal between VCU and BMS1 is incomplete/2(VDDM_C3BMS1CSCFS_flg) -> VDDM_C3BMS1CSCFS_flg/1
  The CAN signal between VCU and CCU1 is discontinuous/2(VDDM_C3CCU1RCCFS_flg) -> VDDM_C3CCU1RCCFS_flg/1
  The CAN signal between VCU and CCU1 is incomplete/2(VDDM_C3CCU1CSCFS_flg) -> VDDM_C3CCU1CSCFS_flg/1
  The CAN signal between VCU and ABM1 is discontinuous/3(VDDM_C1ABM1RCCFS_flg) -> VDDM_C1ABM1RCCFS_flg/1
  The CAN signal between VCU and ABM1 is incomplete/3(VDDM_C1ABM1CSCFS_flg) -> VDDM_C1ABM1CSCFS_flg/1

== system ddm/DDM/DDM/PMM/Fault level ==
  task_time_s : Inport
  VPMM_PwrStaSW_enum : Inport  Port=2
  VPMM_PowerSta_enum : Inport  Port=3
  VINP_BMSWarn1_flg : Inport  Port=4
  VINP_BMSWarn2_flg : Inport  Port=5
  VINP_BMSWarn3_flg : Inport  Port=6
  VINP_BMSWarn4_flg : Inport  Port=7
  VINP_BMSWarn5_flg : Inport  Port=8
  VINP_BMSWarn6_flg : Inport  Port=9
  VINP_BMSWarn7_flg : Inport  Port=10
  VINP_BMSWarn8_flg : Inport  Port=11
  VINP_DCDCFaultSta_enum : Inport  Port=12
  VPMM_DrivetrainSelect_enum : Inport  Port=13
  VDDM_C3BMS6LCCFS_flg : Inport  Port=14
  VDDM_C3CCU2LCCFS_flg : Inport  Port=15
  VDDM_MCUNF1NoComCFS_flg : Inport  Port=16
  VDDM_MCUNR1NoComCFS_flg : Inport  Port=17
  VINP_MCUWarnFNidec_enum : Inport  Port=18
  VINP_MCUWarnRNidec_enum : Inport  Port=19
  VINP_OBCFaultSta_enum : Inport  Port=20
  DTC_clear_request : Inport  Port=21
  No_CAN3_BUS_OFF : Inport  Port=22
  VDDM_C3CCU2RCCFS_flg : Inport  Port=23
  VDDM_C3CCU2CSCFS_flg : Inport  Port=24
  VDDM_MCUNR1RCErrCFS_flg : Inport  Port=25
  VDDM_MCUNR1CSErrCFS_flg : Inport  Port=26
  VDDM_MCUNF1RCErrCFS_flg : Inport  Port=27
  VDDM_MCUNF1CSErrCFS_flg : Inport  Port=28
  VDDM_C3BMS6RCCFS_flg : Inport  Port=29
  VDDM_C3BMS6CSCFS_flg : Inport  Port=30
  No_CAN1_BUS_OFF : Inport  Port=31
  VDDM_ESC1SigErr_flg : Inport  Port=32
  VDDM_ESC5SigErr_flg : Inport  Port=33
  ZoneFrMalfunLevel_enum : Inport  Port=34
  VDDM_FrVCUNoComCFS_flg : Inport  Port=35
  VINP_ShifterFailsta_enum : Inport  Port=36
  VDDM_Shifter1NoComCFS_flg : Inport  Port=37
  VDDM_Shifter1RCErrCFS_flg : Inport  Port=38
  VDDM_Shifter1CSErrCFS_flg : Inport  Port=39
  VINP_ZoneDrMalfunLevel_enum : Inport  Port=40
  No_CAN4_BUS_OFF : Inport  Port=41
  VDDM_DrVCUNoComCFS_flg : Inport  Port=42
  Fault level 1 subsystem error : Subsystem
  Fault level 2 subsystem error : Subsystem
  Fault level 3 subsystem error : Subsystem
  Fault level 4 subsystem error1 : Subsystem
  VDDM_Lv1ErrDTC_raw32 : Outport
  VDDM_Lv2ErrDTC_raw32 : Outport  Port=2
  VDDM_Lv3ErrDTC_raw32 : Outport  Port=3
  VDDM_Lv4ErrDTC_raw32 : Outport  Port=4
  VDDM_Lv1ErrCFS_flg : Outport  Port=5
  VDDM_Lv2ErrCFS_flg : Outport  Port=6
  VDDM_Lv3ErrCFS_flg : Outport  Port=7
  VDDM_Lv4ErrCFS_flg : Outport  Port=8
  wires:
  [No_CAN3_BUS_OFF] -> Fault level 4 subsystem error1/8(No_CAN3_BUS_OFF)
  [DTC_clear_request] -> Fault level 4 subsystem error1/7(DTC_clear_request)
  [DTC_clear_request] -> Fault level 3 subsystem error/11(DTC_clear_request)
  [No_CAN3_BUS_OFF] -> Fault level 3 subsystem error/12(No_CAN3_BUS_OFF)
  [No_CAN3_BUS_OFF] -> Fault level 2 subsystem error/15(No_CAN3_BUS_OFF)
  [DTC_clear_request] -> Fault level 2 subsystem error/14(DTC_clear_request)
  [DTC_clear_request] -> Fault level 1 subsystem error/16(DTC_clear_request)
  [No_CAN3_BUS_OFF] -> Fault level 1 subsystem error/17(No_CAN3_BUS_OFF)
  DTC_clear_request/1 -> [DTC_clear_request]
  No_CAN3_BUS_OFF/1 -> [No_CAN3_BUS_OFF]
  [VINP_MCUWarnRNidec_enum] -> Fault level 1 subsystem error/13(VINP_MCUWarnRNidec_enum)
  [VINP_MCUWarnFNidec_enum] -> Fault level 1 subsystem error/12(VINP_MCUWarnFNidec_enum)
  [VINP_MCUWarnFNidec_enum] -> Fault level 3 subsystem error/8(VINP_MCUWarnFNidec_enum)
  [VINP_MCUWarnRNidec_enum] -> Fault level 3 subsystem error/9(VINP_MCUWarnRNidec_enum)
  [VPMM_DrivetrainSelect_enum] -> Fault level 3 subsystem error/10(VPMM_DrivetrainSelect_enum)
  [VINP_MCUWarnRNidec_enum] -> Fault level 2 subsystem error/12(VINP_MCUWarnRNidec_enum)
  [VINP_MCUWarnFNidec_enum] -> Fault level 2 subsystem error/11(VINP_MCUWarnFNidec_enum)
  [VPMM_DrivetrainSelect_enum] -> Fault level 2 subsystem error/13(VPMM_DrivetrainSelect_enum)
  [VINP_OBCFaultSta_enum] -> Fault level 1 subsystem error/14(VINP_OBCFaultSta_enum)
  VINP_OBCFaultSta_enum/1 -> [VINP_OBCFaultSta_enum]
  VINP_MCUWarnRNidec_enum/1 -> [VINP_MCUWarnRNidec_enum]
  VINP_MCUWarnFNidec_enum/1 -> [VINP_MCUWarnFNidec_enum]
  [VDDM_C3CCU2LCCFS_flg] -> Fault level 2 subsystem error/5(VDDM_C3CCU2LCCFS_flg)
  [VDDM_C3CCU2LCCFS_flg] -> Fault level 1 subsystem error/5(VDDM_C3CCU2LCCFS_flg)
  VDDM_C3CCU2LCCFS_flg/1 -> [VDDM_C3CCU2LCCFS_flg]
  [VDDM_C3BMS6LCCFS_flg] -> Fault level 4 subsystem error1/4(VDDM_C3BMS6LCCFS_flg)
  [VDDM_C3BMS6LCCFS_flg] -> Fault level 3 subsystem error/4(VDDM_C3BMS6LCCFS_flg)
  [VDDM_MCUNR1NoComCFS_flg] -> Fault level 3 subsystem error/6(VDDM_MCUNR1NoComCFS_flg)
  [VDDM_MCUNF1NoComCFS_flg] -> Fault level 3 subsystem error/5(VDDM_MCUNF1NoComCFS_flg)
  [VDDM_MCUNF1NoComCFS_flg] -> Fault level 2 subsystem error/6(VDDM_MCUNF1NoComCFS_flg)
  [VDDM_MCUNR1NoComCFS_flg] -> Fault level 2 subsystem error/7(VDDM_MCUNR1NoComCFS_flg)
  [VDDM_MCUNF1NoComCFS_flg] -> Fault level 1 subsystem error/6(VDDM_MCUNF1NoComCFS_flg)
  [VDDM_MCUNR1NoComCFS_flg] -> Fault level 1 subsystem error/7(VDDM_MCUNR1NoComCFS_flg)
  VDDM_MCUNF1NoComCFS_flg/1 -> [VDDM_MCUNF1NoComCFS_flg]
  VDDM_MCUNR1NoComCFS_flg/1 -> [VDDM_MCUNR1NoComCFS_flg]
  [VDDM_C3BMS6LCCFS_flg] -> Fault level 2 subsystem error/4(VDDM_C3BMS6LCCFS_flg)
  [VDDM_C3BMS6LCCFS_flg] -> Fault level 1 subsystem error/4(VDDM_C3BMS6LCCFS_flg)
  VDDM_C3BMS6LCCFS_flg/1 -> [VDDM_C3BMS6LCCFS_flg]
  [task_time_s] -> Fault level 4 subsystem error1/1(task_time_s)
  [VPMM_DrivetrainSelect_enum] -> Fault level 1 subsystem error/15(VPMM_DrivetrainSelect_enum)
  VPMM_DrivetrainSelect_enum/1 -> [VPMM_DrivetrainSelect_enum]
  [VPMM_PowerSta_enum] -> Fault level 3 subsystem error/2(VPMM_PowerSta_enum)
  [VPMM_PwrStaSW_enum] -> Fault level 3 subsystem error/3(VPMM_PwrStaSW_enum)
  [task_time_s] -> Fault level 3 subsystem error/1(task_time_s)
  [VINP_DCDCFaultSta_enum] -> Fault level 1 subsystem error/11(VINP_DCDCFaultSta_enum)
  [VINP_DCDCFaultSta_enum] -> Fault level 2 subsystem error/10(VINP_DCDCFaultSta_enum)
  VINP_DCDCFaultSta_enum/1 -> [VINP_DCDCFaultSta_enum]
  [task_time_s] -> Fault level 2 subsystem error/1(task_time_s)
  [VPMM_PwrStaSW_enum] -> Fault level 2 subsystem error/3(VPMM_PwrStaSW_enum)
  [VPMM_PowerSta_enum] -> Fault level 2 subsystem error/2(VPMM_PowerSta_enum)
  [VPMM_PowerSta_enum] -> Fault level 1 subsystem error/2(VPMM_PowerSta_enum)
  [VPMM_PwrStaSW_enum] -> Fault level 1 subsystem error/3(VPMM_PwrStaSW_enum)
  [task_time_s] -> Fault level 1 subsystem error/1(task_time_s)
  VPMM_PowerSta_enum/1 -> [VPMM_PowerSta_enum]
  VPMM_PwrStaSW_enum/1 -> [VPMM_PwrStaSW_enum]
  task_time_s/1 -> [task_time_s]
  [VDDM_C3CCU2RCCFS_flg] -> Fault level 1 subsystem error/18(VDDM_C3CCU2RCCFS_flg)
  [VDDM_C3CCU2CSCFS_flg] -> Fault level 1 subsystem error/19(VDDM_C3CCU2CSCFS_flg)
  [VDDM_MCUNR1RCErrCFS_flg] -> Fault level 1 subsystem error/20(VDDM_MCUNR1RCErrCFS_flg)
  [VDDM_MCUNR1CSErrCFS_flg] -> Fault level 1 subsystem error/21(VDDM_MCUNR1CSErrCFS_flg)
  [VDDM_MCUNF1RCErrCFS_flg] -> Fault level 1 subsystem error/22(VDDM_MCUNF1RCErrCFS_flg)
  [VDDM_MCUNF1CSErrCFS_flg] -> Fault level 1 subsystem error/23(VDDM_MCUNF1CSErrCFS_flg)
  [VDDM_C3BMS6RCCFS_flg] -> Fault level 1 subsystem error/24(VDDM_C3BMS6RCCFS_flg)
  [VDDM_C3BMS6CSCFS_flg] -> Fault level 1 subsystem error/25(VDDM_C3BMS6CSCFS_flg)
  [No_CAN1_BUS_OFF] -> Fault level 1 subsystem error/26(No_CAN1_BUS_OFF)
  [VDDM_ESC1SigErr_flg] -> Fault level 1 subsystem error/27(VDDM_ESC1SigErr_flg)
  [VDDM_ESC5SigErr_flg] -> Fault level 1 subsystem error/28(VDDM_ESC5SigErr_flg)
  [VINP_ShifterFailsta_enum] -> Fault level 1 subsystem error/29(VINP_ShifterFailsta_enum)
  [VDDM_Shifter1NoComCFS_flg] -> Fault level 1 subsystem error/30(VDDM_Shifter1NoComCFS_flg)
  [VDDM_Shifter1RCErrCFS_flg] -> Fault level 1 subsystem error/31(VDDM_Shifter1RCErrCFS_flg)
  [VDDM_Shifter1CSErrCFS_flg] -> Fault level 1 subsystem error/32(VDDM_Shifter1CSErrCFS_flg)
  [VINP_ZoneDrMalfunLevel_enum] -> Fault level 1 subsystem error/33(VINP_ZoneDrMalfunLevel_enum)
  [No_CAN4_BUS_OFF] -> Fault level 1 subsystem error/34(No_CAN4_BUS_OFF)
  [VDDM_DrVCUNoComCFS_flg] -> Fault level 1 subsystem error/35(VDDM_DrVCUNoComCFS_flg)
  [ZoneFrMalfunLevel_enum] -> Fault level 1 subsystem error/36(ZoneFrMalfunLevel_enum)
  [VDDM_FrVCUNoComCFS_flg] -> Fault level 1 subsystem error/37(VDDM_FrVCUNoComCFS_flg)
  [VDDM_C3CCU2RCCFS_flg] -> Fault level 2 subsystem error/16(VDDM_C3CCU2RCCFS_flg)
  [VDDM_C3CCU2CSCFS_flg] -> Fault level 2 subsystem error/17(VDDM_C3CCU2CSCFS_flg)
  [VDDM_MCUNR1RCErrCFS_flg] -> Fault level 2 subsystem error/18(VDDM_MCUNR1RCErrCFS_flg)
  [VDDM_MCUNR1CSErrCFS_flg] -> Fault level 2 subsystem error/19(VDDM_MCUNR1CSErrCFS_flg)
  [VDDM_MCUNF1RCErrCFS_flg] -> Fault level 2 subsystem error/20(VDDM_MCUNF1RCErrCFS_flg)
  [VDDM_MCUNF1CSErrCFS_flg] -> Fault level 2 subsystem error/21(VDDM_MCUNF1CSErrCFS_flg)
  [VDDM_C3BMS6RCCFS_flg] -> Fault level 2 subsystem error/22(VDDM_C3BMS6RCCFS_flg)
  [VDDM_C3BMS6CSCFS_flg] -> Fault level 2 subsystem error/23(VDDM_C3BMS6CSCFS_flg)
  [VINP_ZoneDrMalfunLevel_enum] -> Fault level 2 subsystem error/24(ZoneDrMalfunLevel_enum)
  [No_CAN4_BUS_OFF] -> Fault level 2 subsystem error/25(No_CAN4_BUS_OFF)
  [VDDM_DrVCUNoComCFS_flg] -> Fault level 2 subsystem error/26(VDDM_DrVCUNoComCFS_flg)
  [ZoneFrMalfunLevel_enum] -> Fault level 2 subsystem error/27(ZoneFrMalfunLevel_enum)
  [VDDM_FrVCUNoComCFS_flg] -> Fault level 2 subsystem error/28(VDDM_FrVCUNoComCFS_flg)
  [VDDM_MCUNR1RCErrCFS_flg] -> Fault level 3 subsystem error/13(VDDM_MCUNR1RCErrCFS_flg)
  [VDDM_MCUNR1CSErrCFS_flg] -> Fault level 3 subsystem error/14(VDDM_MCUNR1CSErrCFS_flg)
  [VDDM_MCUNF1RCErrCFS_flg] -> Fault level 3 subsystem error/15(VDDM_MCUNF1RCErrCFS_flg)
  [VDDM_MCUNF1CSErrCFS_flg] -> Fault level 3 subsystem error/16(VDDM_MCUNF1CSErrCFS_flg)
  [VDDM_C3BMS6RCCFS_flg] -> Fault level 3 subsystem error/17(VDDM_C3BMS6RCCFS_flg)
  [VDDM_C3BMS6CSCFS_flg] -> Fault level 3 subsystem error/18(VDDM_C3BMS6CSCFS_flg)
  [VINP_ZoneDrMalfunLevel_enum] -> Fault level 3 subsystem error/19(ZoneDrMalfunLevel_enum)
  [No_CAN4_BUS_OFF] -> Fault level 3 subsystem error/20(No_CAN4_BUS_OFF)
  [VDDM_DrVCUNoComCFS_flg] -> Fault level 3 subsystem error/21(VDDM_DrVCUNoComCFS_flg)
  [ZoneFrMalfunLevel_enum] -> Fault level 3 subsystem error/22(ZoneFrMalfunLevel_enum)
  [VDDM_FrVCUNoComCFS_flg] -> Fault level 3 subsystem error/23(VDDM_FrVCUNoComCFS_flg)
  [VPMM_PwrStaSW_enum] -> Fault level 4 subsystem error1/3(VPMM_PwrStaSW_enum)
  [VPMM_PowerSta_enum] -> Fault level 4 subsystem error1/2(VPMM_PowerSta_enum)
  [VDDM_C3BMS6RCCFS_flg] -> Fault level 4 subsystem error1/9(VDDM_C3BMS6RCCFS_flg)
  [VDDM_C3BMS6CSCFS_flg] -> Fault level 4 subsystem error1/10(VDDM_C3BMS6CSCFS_flg)
  [VINP_ZoneDrMalfunLevel_enum] -> Fault level 4 subsystem error1/11(ZoneDrMalfunLevel_enum)
  [No_CAN4_BUS_OFF] -> Fault level 4 subsystem error1/12(No_CAN4_BUS_OFF)
  [VDDM_DrVCUNoComCFS_flg] -> Fault level 4 subsystem error1/13(VDDM_DrVCUNoComCFS_flg)
  [ZoneFrMalfunLevel_enum] -> Fault level 4 subsystem error1/14(ZoneFrMalfunLevel_enum)
  [VDDM_FrVCUNoComCFS_flg] -> Fault level 4 subsystem error1/15(VDDM_FrVCUNoComCFS_flg)
  VINP_BMSWarn1_flg/1 -> [VINP_BMSWarn1_flg]
  VINP_BMSWarn2_flg/1 -> [VINP_BMSWarn2_flg]
  VINP_BMSWarn3_flg/1 -> [VINP_BMSWarn3_flg]
  VINP_BMSWarn4_flg/1 -> [VINP_BMSWarn4_flg]
  VINP_BMSWarn5_flg/1 -> [VINP_BMSWarn5_flg]
  VINP_BMSWarn6_flg/1 -> [VINP_BMSWarn6_flg]
  VINP_BMSWarn7_flg/1 -> [VINP_BMSWarn7_flg]
  VINP_BMSWarn8_flg/1 -> [VINP_BMSWarn8_flg]
  [VINP_BMSWarn1_flg] -> Fault level 1 subsystem error/8(VINP_BMSWarn1_flg)
  [VINP_BMSWarn2_flg] -> Fault level 1 subsystem error/9(VINP_BMSWarn2_flg)
  [VINP_BMSWarn3_flg] -> Fault level 1 subsystem error/10(VINP_BMSWarn3_flg)
  [VINP_BMSWarn4_flg] -> Fault level 2 subsystem error/8(VINP_BMSWarn4_flg)
  [VINP_BMSWarn5_flg] -> Fault level 2 subsystem error/9(VINP_BMSWarn5_flg)
  [VINP_BMSWarn6_flg] -> Fault level 3 subsystem error/7(VINP_BMSWarn6_flg)
  [VINP_BMSWarn7_flg] -> Fault level 4 subsystem error1/5(VINP_BMSWarn7_flg)
  [VINP_BMSWarn8_flg] -> Fault level 4 subsystem error1/6(VINP_BMSWarn8_flg)
  Fault level 1 subsystem error/1(VDDM_Lv1ErrCFS_flg) -> [VDDM_Lv1ErrCFS_flg]
  Fault level 1 subsystem error/2(VDDM_Lv1ErrDTC_raw32) -> [VDDM_Lv1ErrDTC_raw32]
  Fault level 2 subsystem error/1(VDDM_Lv2ErrCFS_flg) -> [VDDM_Lv2ErrCFS_flg]
  Fault level 3 subsystem error/1(VDDM_Lv3ErrCFS_flg) -> [VDDM_Lv3ErrCFS_flg]
  Fault level 4 subsystem error1/1(VDDM_Lv4ErrCFS_flg) -> [VDDM_Lv4ErrCFS_flg]
  Fault level 2 subsystem error/2(VDDM_Lv2ErrDTC_raw32) -> [VDDM_Lv2ErrDTC_raw32]
  Fault level 3 subsystem error/2(VDDM_Lv3ErrDTC_raw32) -> [VDDM_Lv3ErrDTC_raw32]
  Fault level 4 subsystem error1/2(VDDM_Lv4ErrDTC_raw32) -> [VDDM_Lv4ErrDTC_raw32]
  [VDDM_Lv1ErrDTC_raw32] -> VDDM_Lv1ErrDTC_raw32/1
  [VDDM_Lv2ErrDTC_raw32] -> VDDM_Lv2ErrDTC_raw32/1
  [VDDM_Lv3ErrDTC_raw32] -> VDDM_Lv3ErrDTC_raw32/1
  [VDDM_Lv4ErrDTC_raw32] -> VDDM_Lv4ErrDTC_raw32/1
  [VDDM_Lv1ErrCFS_flg] -> VDDM_Lv1ErrCFS_flg/1
  [VDDM_Lv2ErrCFS_flg] -> VDDM_Lv2ErrCFS_flg/1
  [VDDM_Lv3ErrCFS_flg] -> VDDM_Lv3ErrCFS_flg/1
  [VDDM_Lv4ErrCFS_flg] -> VDDM_Lv4ErrCFS_flg/1
  VDDM_MCUNF1RCErrCFS_flg/1 -> [VDDM_MCUNF1RCErrCFS_flg]
  VDDM_C3BMS6RCCFS_flg/1 -> [VDDM_C3BMS6RCCFS_flg]
  VDDM_MCUNR1RCErrCFS_flg/1 -> [VDDM_MCUNR1RCErrCFS_flg]
  VDDM_MCUNR1CSErrCFS_flg/1 -> [VDDM_MCUNR1CSErrCFS_flg]
  VDDM_C3CCU2CSCFS_flg/1 -> [VDDM_C3CCU2CSCFS_flg]
  VDDM_C3CCU2RCCFS_flg/1 -> [VDDM_C3CCU2RCCFS_flg]
  VDDM_MCUNF1CSErrCFS_flg/1 -> [VDDM_MCUNF1CSErrCFS_flg]
  VDDM_ESC5SigErr_flg/1 -> [VDDM_ESC5SigErr_flg]
  VDDM_ESC1SigErr_flg/1 -> [VDDM_ESC1SigErr_flg]
  No_CAN1_BUS_OFF/1 -> [No_CAN1_BUS_OFF]
  VDDM_C3BMS6CSCFS_flg/1 -> [VDDM_C3BMS6CSCFS_flg]
  ZoneFrMalfunLevel_enum/1 -> [ZoneFrMalfunLevel_enum]
  VDDM_FrVCUNoComCFS_flg/1 -> [VDDM_FrVCUNoComCFS_flg]
  No_CAN4_BUS_OFF/1 -> [No_CAN4_BUS_OFF]
  VINP_ZoneDrMalfunLevel_enum/1 -> [VINP_ZoneDrMalfunLevel_enum]
  VDDM_DrVCUNoComCFS_flg/1 -> [VDDM_DrVCUNoComCFS_flg]
  VDDM_Shifter1NoComCFS_flg/1 -> [VDDM_Shifter1NoComCFS_flg]
  VDDM_Shifter1RCErrCFS_flg/1 -> [VDDM_Shifter1RCErrCFS_flg]
  VINP_ShifterFailsta_enum/1 -> [VINP_ShifterFailsta_enum]
  VDDM_Shifter1CSErrCFS_flg/1 -> [VDDM_Shifter1CSErrCFS_flg]

== system ddm/DDM/DDM/PMM/Key authentication failed ==
  note: Diagnostics and Fault Handling
  note: Test Pass Criteria
  note: Release Condition After Decision
  note: Test Detection Criteria
  task_time_s : Inport
  VPMM_PowerSta_enum : Inport  Port=2
  VPMM_PwrStaSW_enum : Inport  Port=3
  DTC_clear_request : Inport  Port=4
  VDKC_DKCAuthSta_enum : Inport  Port=5
  VINP_CANMsgValidDKC2_flg : Inport  Port=6
  VINP_CANMsgValidDKC1_flg : Inport  Port=7
  Constant1 : Constant  Value=TRUE
  Constant10 : Constant  Value=ENUM_POWERSTA_STANDBY
  Constant12 : Constant  Value=FALSE
  Constant13 : Constant  Value=KDDM_KeyAuthDTC_cnt
  Constant14 : Constant  Value=KDDM_KeyAuthPassTO_s
  Constant17 : Constant  Value=KDDM_KeyAuthPassTO_s
  Constant18 : Constant  Value=KDDM_KeyAuthDTC_cnt
  Constant2 : Constant  Value=ENUM_PWRSTASW_OFF
  Constant22 : Constant  Value=FALSE
  Constant28 : Constant  Value=ENUM_PWRSTASW_OFF
  Constant30 : Constant  Value=KDDM_KeyAuthDiagnosisOffSW_flg
  Constant31 : Constant  Value=ENUM_POWERSTA_OFF
  Constant6 : Constant  Value=ZERO_INT
  Constant9 : Constant  Value=KDDM_KeyAuthDetTO_s
  DTC_Couter1 : hcu_lib/Basic_Blocks/DTC_Couter
  DTC_Info : hcu_lib/Basic_Blocks/DTC_Info
  Equal1 : RelationalOperator  Operator=~=  OutDataTypeStr=boolean  RndMeth=Simplest
  Equal10 : RelationalOperator  Operator===  OutDataTypeStr=boolean  RndMeth=Simplest
  Equal2 : RelationalOperator  Operator=~=  OutDataTypeStr=boolean  RndMeth=Simplest
  Equal8 : RelationalOperator  OutDataTypeStr=boolean  RndMeth=Simplest
  Equal9 : RelationalOperator  Operator===  OutDataTypeStr=boolean  RndMeth=Simplest
  Logical Operator : Logic  Inputs=3  AllPortsSameDT=off  OutDataTypeStr=boolean
  Logical Operator1 : Logic  Inputs=3  AllPortsSameDT=off  OutDataTypeStr=boolean
  Logical Operator16 : Logic  Operator=OR  Inputs=4  AllPortsSameDT=off  OutDataTypeStr=boolean
  Logical Operator17 : Logic  AllPortsSameDT=off  OutDataTypeStr=boolean
  Logical Operator21 : Logic  Operator=NOT  AllPortsSameDT=off  OutDataTypeStr=boolean
  Relational Operator1 : RelationalOperator  Operator=>  OutDataTypeStr=boolean  RndMeth=Simplest
  Switch1 : Switch  Criteria=u2 ~= 0
  Switch8 : Switch  Criteria=u2 ~= 0
  Switch9 : Switch  Criteria=u2 ~= 0
  Terminator : Terminator
  Test Detection Criteria1 : hcu_lib/Basic_Blocks/Test Detection Criteria
  Timer2 : hcu_lib/Basic_Blocks/Timer
  Unit Delay1 : UnitDelay  SampleTime=-1  HasFrameUpgradeWarning=on
  VDDM_KeyAuthDTC_raw32 : Outport
  VDDM_KeyAuthCFS_flg : Outport  Port=2
  wires:
  [VDDM_KeyAuthCFS_flg] -> VDDM_KeyAuthCFS_flg/1
  [VDDM_KeyAuthPass_flg] -> Logical Operator16/3
  [VPMM_PwrStaSW_enum] -> Equal1/1
  Constant28/1 -> Equal1/2
  Test Detection Criteria1/1 -> [VDDM_KeyAuthDet_flg]  "VDDM_KeyAuthDet_flg"
  [VDKC_DKCAuthSta_enum] -> Switch8/1
  Equal9/1 -> Logical Operator17/1
  Constant10/1 -> Equal10/2
  Constant17/1 -> Equal8/2
  Constant14/1 -> Timer2/4
  Constant22/1 -> Switch9/1
  [VPMM_PowerSta_enum] -> Equal10/1
  [VDDM_KeyAuthCFSRls_flg] -> DTC_Couter1/2
  Constant18/1 -> DTC_Couter1/3
  DTC_Couter1/1 -> [VDDM_KeyAuthCFS_flg]  "VDDM_KeyAuthCFS_flg"
  Relational Operator1/1 -> Terminator/1  "VDDM_KeyAuthDFS_flg"
  Timer2/1 -> Equal8/1
  Switch9/1 -> Test Detection Criteria1/1
  Constant12/1 -> Switch1/3
  Logical Operator21/1 -> Timer2/1
  Equal10/1 -> Logical Operator17/2
  DTC_Couter1/2 -> Relational Operator1/1  "VDDM_KeyAuthDTC_cnt"
  Constant31/1 -> Equal9/2
  Logical Operator17/1 -> Logical Operator16/1
  [DTC_clear_request] -> Logical Operator16/2
  [task_time_s] -> Timer2/3
  Constant30/1 -> Logical Operator16/4
  Constant1/1 -> Switch8/3
  [VDDM_KeyAuthCFSRls_flg] -> Switch9/2
  Switch1/1 -> Switch9/3
  [task_time_s] -> Test Detection Criteria1/2
  [VPMM_PowerSta_enum] -> Unit Delay1/1
  Switch8/1 -> Logical Operator21/1, Timer2/2
  Equal8/1 -> [VDDM_KeyAuthPass_flg]  "VDDM_KeyAuthPass_flg"
  Constant6/1 -> Relational Operator1/2
  Unit Delay1/1 -> Equal9/1
  Constant9/1 -> Test Detection Criteria1/4
  [VDDM_KeyAuthDet_flg] -> DTC_Couter1/1
  Logical Operator16/1 -> [VDDM_KeyAuthCFSRls_flg]  "VDDM_KeyAuthCFSRls_flg"
  Constant13/1 -> Test Detection Criteria1/3
  VPMM_PowerSta_enum/1 -> [VPMM_PowerSta_enum]
  VPMM_PwrStaSW_enum/1 -> [VPMM_PwrStaSW_enum]
  task_time_s/1 -> [task_time_s]
  VDKC_DKCAuthSta_enum/1 -> [VDKC_DKCAuthSta_enum]
  DTC_clear_request/1 -> [DTC_clear_request]
  [VDDM_KeyAuthPass_flg] -> DTC_Info/2
  [VDDM_KeyAuthCFS_flg] -> DTC_Info/3
  DTC_Info/1 -> VDDM_KeyAuthDTC_raw32/1  "VDDM_KeyAuthDTC_raw32"
  [VDDM_KeyAuthDet_flg] -> DTC_Info/1
  [DTC_clear_request] -> DTC_Info/4
  [VDKC_DKCAuthSta_enum] -> Switch1/1
  VINP_CANMsgValidDKC2_flg/1 -> [VINP_CANMsgValidDKC2_flg]
  VINP_CANMsgValidDKC1_flg/1 -> [VINP_CANMsgValidDKC1_flg]
  Logical Operator/1 -> Switch1/2
  Equal1/1 -> Logical Operator/1
  [VINP_CANMsgValidDKC1_flg] -> Logical Operator/2
  [VINP_CANMsgValidDKC2_flg] -> Logical Operator/3
  [VINP_CANMsgValidDKC1_flg] -> Logical Operator1/2
  Equal2/1 -> Logical Operator1/1
  [VPMM_PwrStaSW_enum] -> Equal2/1
  Logical Operator1/1 -> Switch8/2
  Constant2/1 -> Equal2/2
  [VINP_CANMsgValidDKC2_flg] -> Logical Operator1/3

== system ddm/DDM/DDM/PMM/LV ==
  task_time_s : Inport
  VPMM_PwrStaSW_enum : Inport  Port=2
  VPMM_PowerSta_enum : Inport  Port=3
  VINP_LVBattDet12V_V : Inport  Port=4
  VINP_CANMsgValidBMS5_flg : Inport  Port=5
  DTC_clear_request : Inport  Port=6
  VDDM_AuxBattVolV_V : Inport  Port=7
  Initial LV battery voltage too low : Subsystem
  LV analog input error : Subsystem
  LV power supply voltage too high : Subsystem
  LV power supply voltage too low : Subsystem
  Logical Operator : Logic  Operator=OR  Inputs=4  AllPortsSameDT=off  OutDataTypeStr=boolean
  VDDM_IniLVLoDTC_raw32 : Outport
  VDDM_LVSupLoDTC_raw32 : Outport  Port=2
  VDDM_LVSupHiDTC_raw32 : Outport  Port=3
  VDDM_LVInErrDTC_raw32 : Outport  Port=4
  VDDM_IniLVLoCFS_flg : Outport  Port=5
  VDDM_LVSupLoCFS_flg : Outport  Port=6
  VDDM_LVSupHiCFS_flg : Outport  Port=7
  VDDM_LVInErrCFS_flg : Outport  Port=8
  VDDM_PMMBattErr_flg : Outport  Port=9
  wires:
  DTC_clear_request/1 -> [DTC_clear_request]
  [DTC_clear_request] -> LV power supply voltage too high/6(DTC_clear_request)
  [VINP_LVBattDet12V_V] -> LV power supply voltage too high/4(VINP_LVBattDet12V_V)
  [VPMM_PowerSta_enum] -> LV power supply voltage too high/2(VPMM_PowerSta_enum)
  [VINP_CANMsgValidBMS5_flg] -> LV power supply voltage too high/5(VINP_CANMsgValidBMS5_flg)
  [VPMM_PwrStaSW_enum] -> LV power supply voltage too high/3(VPMM_PwrStaSW_enum)
  [task_time_s] -> LV power supply voltage too high/1(task_time_s)
  [VINP_LVBattDet12V_V] -> LV power supply voltage too low/4(VINP_LVBattDet12V_V)
  [VINP_CANMsgValidBMS5_flg] -> LV power supply voltage too low/5(VINP_CANMsgValidBMS5_flg)
  [task_time_s] -> LV power supply voltage too low/1(task_time_s)
  [DTC_clear_request] -> LV power supply voltage too low/6(DTC_clear_request)
  [VPMM_PwrStaSW_enum] -> LV power supply voltage too low/3(VPMM_PwrStaSW_enum)
  [VPMM_PowerSta_enum] -> LV power supply voltage too low/2(VPMM_PowerSta_enum)
  [VPMM_PowerSta_enum] -> Initial LV battery voltage too low/2(VPMM_PowerSta_enum)
  [VPMM_PwrStaSW_enum] -> Initial LV battery voltage too low/3(VPMM_PwrStaSW_enum)
  [DTC_clear_request] -> Initial LV battery voltage too low/6(DTC_clear_request)
  [VINP_CANMsgValidBMS5_flg] -> Initial LV battery voltage too low/5(VINP_CANMsgValidBMS5_flg)
  [VINP_LVBattDet12V_V] -> Initial LV battery voltage too low/4(VINP_LVBattDet12V_V)
  [task_time_s] -> Initial LV battery voltage too low/1(task_time_s)
  VINP_LVBattDet12V_V/1 -> [VINP_LVBattDet12V_V]
  task_time_s/1 -> [task_time_s]
  VPMM_PwrStaSW_enum/1 -> [VPMM_PwrStaSW_enum]
  VPMM_PowerSta_enum/1 -> [VPMM_PowerSta_enum]
  Initial LV battery voltage too low/1(VDDM_IniLVLoDTC_raw32) -> VDDM_IniLVLoDTC_raw32/1  "VDDM_IniLVLoDTC_raw32"
  LV power supply voltage too low/1(VDDM_LVSupLoDTC_raw32) -> VDDM_LVSupLoDTC_raw32/1  "VDDM_LVSupLoDTC_raw32"
  LV power supply voltage too high/1(VDDM_LVSupHiDTC_raw32) -> VDDM_LVSupHiDTC_raw32/1  "VDDM_LVSupHiDTC_raw32"
  Initial LV battery voltage too low/2(VDDM_IniLVLoCFS_flg) -> [VDDM_IniLVLoCFS_flg]
  LV power supply voltage too low/2(VDDM_LVSupLoCFS_flg) -> [VDDM_LVSupLoCFS_flg]
  LV power supply voltage too high/2(VDDM_LVSupHiCFS_flg) -> [VDDM_LVSupHiCFS_flg]
  [VPMM_PowerSta_enum] -> LV analog input error/2(VPMM_PowerSta_enum)
  LV analog input error/2(VDDM_LVInErrCFS_flg) -> [VDDM_LVInErrCFS_flg]
  [VDDM_AuxBattVolV_V] -> LV analog input error/6(VDDM_AuxBattVolV_V)
  [VINP_LVBattDet12V_V] -> LV analog input error/3(VINP_LVBattDet12V_V)
  [task_time_s] -> LV analog input error/1(task_time_s)
  [DTC_clear_request] -> LV analog input error/5(DTC_clear_request)
  [VINP_CANMsgValidBMS5_flg] -> LV analog input error/4(VINP_CANMsgValidBMS5_flg)
  LV analog input error/1(VDDM_LVInErrDTC_raw32) -> VDDM_LVInErrDTC_raw32/1
  [VDDM_IniLVLoCFS_flg] -> VDDM_IniLVLoCFS_flg/1
  [VDDM_LVSupLoCFS_flg] -> VDDM_LVSupLoCFS_flg/1
  [VDDM_LVSupHiCFS_flg] -> VDDM_LVSupHiCFS_flg/1
  [VDDM_LVInErrCFS_flg] -> VDDM_LVInErrCFS_flg/1
  VDDM_AuxBattVolV_V/1 -> [VDDM_AuxBattVolV_V]
  VINP_CANMsgValidBMS5_flg/1 -> [VINP_CANMsgValidBMS5_flg]
  [VDDM_IniLVLoCFS_flg] -> Logical Operator/1
  [VDDM_LVSupLoCFS_flg] -> Logical Operator/2
  [VDDM_LVSupHiCFS_flg] -> Logical Operator/3
  [VDDM_LVInErrCFS_flg] -> Logical Operator/4
  Logical Operator/1 -> VDDM_PMMBattErr_flg/1  "VDDM_PMMBattErr_flg"
